simulink model "combined_callback_csv_model"  (R2025b)
settings: Solver=FixedStepDiscrete  StartTime=0.0  StopTime=50  FixedStep=0.1  RelTol=1e-3
PreLoadFcn:
  | callback_preload();
InitFcn:
  | callback_init();
StartFcn:
  | callback_start();
StopFcn:
  | callback_stop();
undefined symbols (not defined in the file or in its folder): amplitude_param, frequency_param
libraries: simulink x1
CloseFcn:
  | callback_close();
settings Model: Creator=KoayXianCong  LastModifiedBy=KoayXianCong

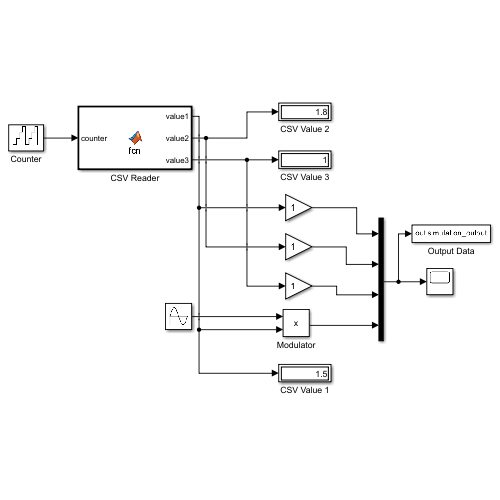
[thumbnail: Simulink's stored preview of the top-level diagram]
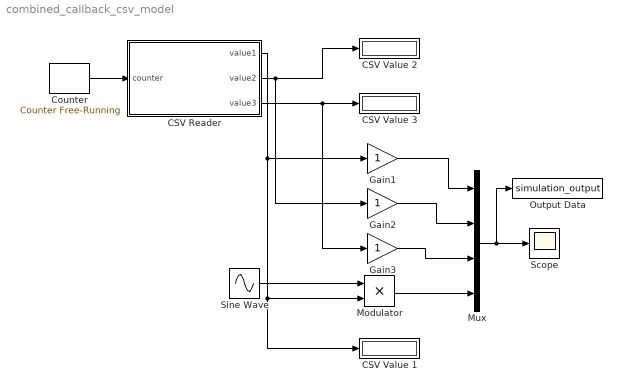
== system combined_callback_csv_model ==
  CSV Reader : MATLAB Function  TreatAsAtomicUnit=on
  CSV Value 1 : Display
  CSV Value 2 : Display
  CSV Value 3 : Display
  Counter : simulink/Sources/Counter Free-Running  NumBits=16  tsamp=-1
  Gain1 : Gain
  Gain2 : Gain
  Gain3 : Gain
  Modulator : Product
  Mux : Mux
  Output Data : ToWorkspace  VariableName=simulation_output  SampleTime=-1
  Scope : Scope
  Sine Wave : Sin  Amplitude=amplitude_param  Frequency=frequency_param  SampleTime=0
  wires:
  Counter/1 -> CSV Reader/1(counter)
  CSV Reader/1(value1) -> CSV Value 1/1, Modulator/2, Gain1/1
  CSV Reader/3(value3) -> Gain3/1, CSV Value 3/1
  CSV Reader/2(value2) -> Gain2/1, CSV Value 2/1
  Sine Wave/1 -> Modulator/1
  Gain1/1 -> Mux/1
  Modulator/1 -> Mux/4
  Gain3/1 -> Mux/3
  Gain2/1 -> Mux/2
  Mux/1 -> Scope/1, Output Data/1

== matlab function combined_callback_csv_model/CSV Reader ==
  data: counter input; value1 output; value2 output; value3 output
function [value1, value2, value3] = fcn(counter)
%% CSV Reader with Counter
% Reads data from input_data.csv based on counter

coder.extrinsic('readtable', 'exist');

% Convert counter to double (Counter block outputs uint16)
counter_double = double(counter);

% Declare persistent variables with explicit types
persistent lastCounter;
persistent data;

if isempty(lastCounter)
    lastCounter = double(0);  % Initialize as double
    data = [1.5, 1.8, 1.0];   % Default values
end

%% Update CSV data every 50 counter steps
if counter_double - lastCounter >= 50
    % Try to read CSV file
    if coder.target('MATLAB')
        if exist('input_data.csv', 'file')
            try
                T = readtable('input_data.csv', 'ReadVariableNames', false);
                if ~isempty(T)
                    data(1) = T{1,1};
                    data(2) = T{1,2};
                    data(3) = T{1,3};
                end
            catch
                % Keep last good data on error
            end
        end
    end
    lastCounter = counter_double;  % Update with double value
end

value1 = data(1);
value2 = data(2);
value3 = data(3);
